simulink model "quadcopterR2Feedback"  (R2022b)
settings: Solver=VariableStepAuto  StartTime=0.0  StopTime=10  RelTol=1e-3
values from neighbouring files (symbols this model uses):
  Az = sys_z.A    [quadcopter_analysis.m]
  Bz = sys_z.B    [quadcopter_analysis.m]
  Cz = sys_z.C    [quadcopter_analysis.m]
  Dz = sys_z.D    [quadcopter_analysis.m]
  K = place(Az,Bz,p)    [quadcopter_analysis.m]
  phi_init = 0.1    [quadcopter_analysis.m]
  psi_init = 0    [quadcopter_analysis.m]
  theta_init = 0    [quadcopter_analysis.m]
  TS = 0.02    [quadcopter_analysis.m]
settings Model: Creator=collinlove  LastModifiedBy=E

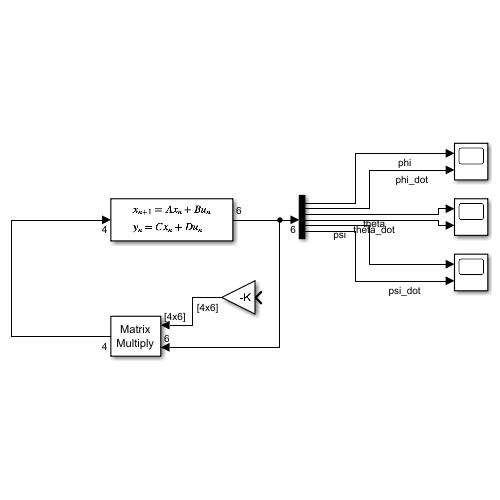
[thumbnail: Simulink's stored preview of the top-level diagram]
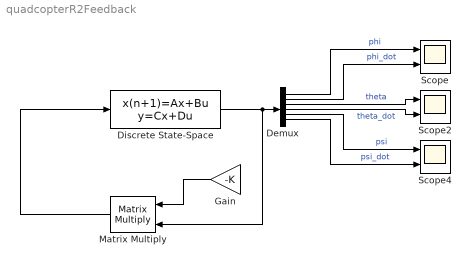
== system quadcopterR2Feedback ==
  Demux : Demux  Outputs=6
  Discrete State-Space : DiscreteStateSpace  A=Az  B=Bz  C=Cz  D=Dz  InitialCondition=[phi_init,0,theta_init,0,psi_init,0]  SampleTime=TS
  Gain : Gain  Gain=-K
  Matrix Multiply : Product  Multiplication=Matrix(*)
  Scope : Scope  NumInputPorts=2
  Scope2 : Scope  NumInputPorts=2
  Scope4 : Scope  NumInputPorts=2
  wires:
  Demux/1 -> Scope/1  "phi"
  Demux/2 -> Scope/2  "phi_dot"
  Demux/3 -> Scope2/1  "theta"
  Demux/4 -> Scope2/2  "theta_dot"
  Demux/5 -> Scope4/1  "psi"
  Demux/6 -> Scope4/2  "psi_dot"
  Discrete State-Space/1 -> Matrix Multiply/2, Demux/1
  Matrix Multiply/1 -> Discrete State-Space/1
  Gain/1 -> Matrix Multiply/1
